simulink model "Forward_Converter_Mathematical_Modelling"  (R2015a)
settings: Solver=ode45  StartTime=0.0  StopTime=0.01  RelTol=1e-3
values from neighbouring files (symbols this model uses):
  C = 19.5e-06    (= 1.95e-05)    [Forward_Converter_Script.m]
  D = 0.416    [Forward_Converter_Script.m]
  Fsw = 400e03    (= 400000)    [Forward_Converter_Script.m]
  L = 12.12e-06    (= 1.212e-05)    [Forward_Converter_Script.m]
  N1 = 2    [Forward_Converter_Script.m]
  N2 = 4    [Forward_Converter_Script.m]
  R = 5    [Forward_Converter_Script.m]
  Vin = 12    [Forward_Converter_Script.m]
settings Model: Creator=Koustubh  LastModifiedBy=Koustubh

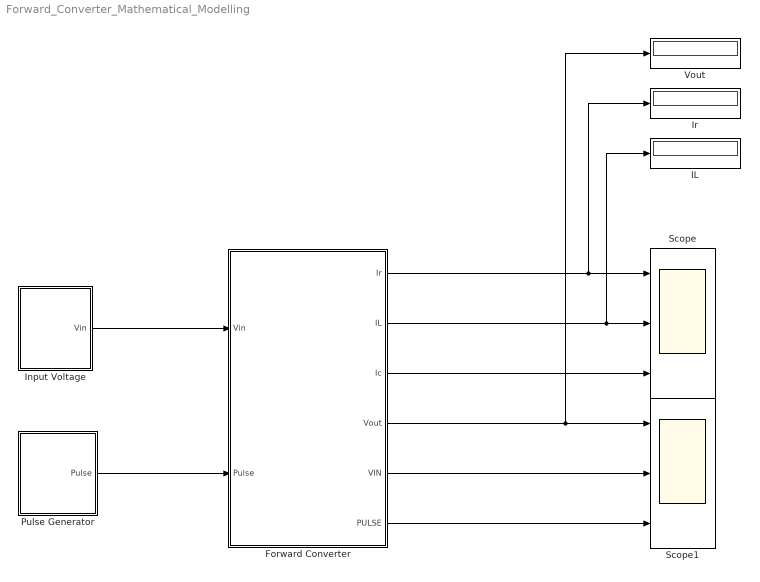
== system Forward_Converter_Mathematical_Modelling ==
  Forward Converter : Subsystem
  IL : Display
  Input Voltage : Subsystem
  Ir : Display
  Pulse Generator : Subsystem
  Scope : Scope  NumInputPorts=3
      settings: YMin=-5~-5~-5  YMax=5~5~5
  Scope1 : Scope  NumInputPorts=3
      settings: YMin=-5~-5~-5  YMax=5~5~5
  Vout : Display
  wires:
  Input Voltage/1(Vin) -> Forward Converter/1(Vin)
  Pulse Generator/1(Pulse) -> Forward Converter/2(Pulse)
  Forward Converter/1(Ir) -> Ir/1, Scope/1
  Forward Converter/3(Ic) -> Scope/3
  Forward Converter/2(IL) -> IL/1, Scope/2
  Forward Converter/4(Vout) -> Vout/1, Scope1/1
  Forward Converter/5(VIN) -> Scope1/2
  Forward Converter/6(PULSE) -> Scope1/3

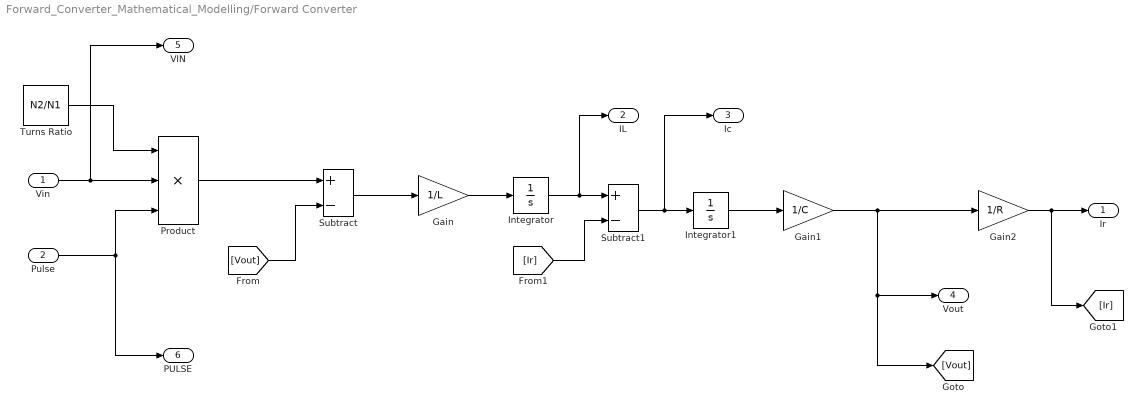
== system Forward_Converter_Mathematical_Modelling/Forward Converter ==
  Vin : Inport
  Pulse : Inport  Port=2
  Gain : Gain  Gain=1/L
  Gain1 : Gain  Gain=1/C
  Gain2 : Gain  Gain=1/R
  Integrator : Integrator
  Integrator1 : Integrator
  Product : Product  Inputs=3
  Subtract : Sum  Inputs=+-
  Subtract1 : Sum  Inputs=+-
  Turns Ratio : Constant  Value=N2/N1
  Ir : Outport
  IL : Outport  Port=2
  Ic : Outport  Port=3
  Vout : Outport  Port=4
  VIN : Outport  Port=5
  PULSE : Outport  Port=6
  wires:
  Vin/1 -> VIN/1, Product/2
  Pulse/1 -> PULSE/1, Product/3
  Turns Ratio/1 -> Product/1
  Product/1 -> Subtract/1
  [Vout] -> Subtract/2
  Subtract/1 -> Gain/1
  Gain/1 -> Integrator/1
  Integrator/1 -> IL/1, Subtract1/1
  [Ir] -> Subtract1/2
  Subtract1/1 -> Ic/1, Integrator1/1
  Integrator1/1 -> Gain1/1
  Gain1/1 -> Vout/1, [Vout], Gain2/1
  Gain2/1 -> [Ir], Ir/1

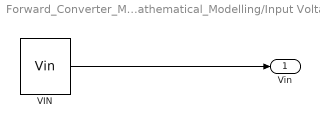
== system Forward_Converter_Mathematical_Modelling/Input Voltage ==
  VIN : Constant  Value=Vin
  Vin : Outport
  wires:
  VIN/1 -> Vin/1

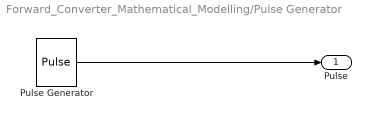
== system Forward_Converter_Mathematical_Modelling/Pulse Generator ==
  Pulse Generator : DiscretePulseGenerator  PulseType=Time based  Period=1/Fsw  PulseWidth=D*100
  Pulse : Outport
  wires:
  Pulse Generator/1 -> Pulse/1
